simulink model "gm_DOA_rearanged"  (R2020b)
settings: Solver=ode4  StartTime=0.0  StopTime=0.25  RelTol=1e-3
undefined symbols (not defined in the file or in its folder): Coeff_han, FFT_LENGTH, Sampling_rate
libraries: dsphdlmathfun x4, dsphdlxfrm x4, simulink x1, hdlsllib x1
settings Model: Creator=tigro  LastModifiedBy=franc
settings OptimizationCC: BlockReduction=off  ConditionallyExecuteInputs=off  DefaultParameterBehavior=Inlined
settings DebuggingCC: AlgebraicLoopMsg=error  InheritedTsInSrcMsg=none  ParameterOverflowMsg=none
settings HardwareCC: ProdBitPerPointer=32  ProdBitPerSizeT=32  ProdBitPerPtrDiffT=32  ProdLargestAtomicFloat=None  ProdIntDivRoundTo=Undefined  ProdEndianess=Unspecified  ProdWordSize=32  ProdHWDeviceType=ASIC/FPGA->ASIC/FPGA  TargetBitPerPointer=64  TargetBitPerSizeT=64  TargetBitPerPtrDiffT=64  TargetLongLongMode=on  TargetIntDivRoundTo=Zero  TargetEndianess=LittleEndian  TargetWordSize=64  TargetHWDeviceType=Custom Processor->MATLAB Host Computer  ProdEqTarget=off

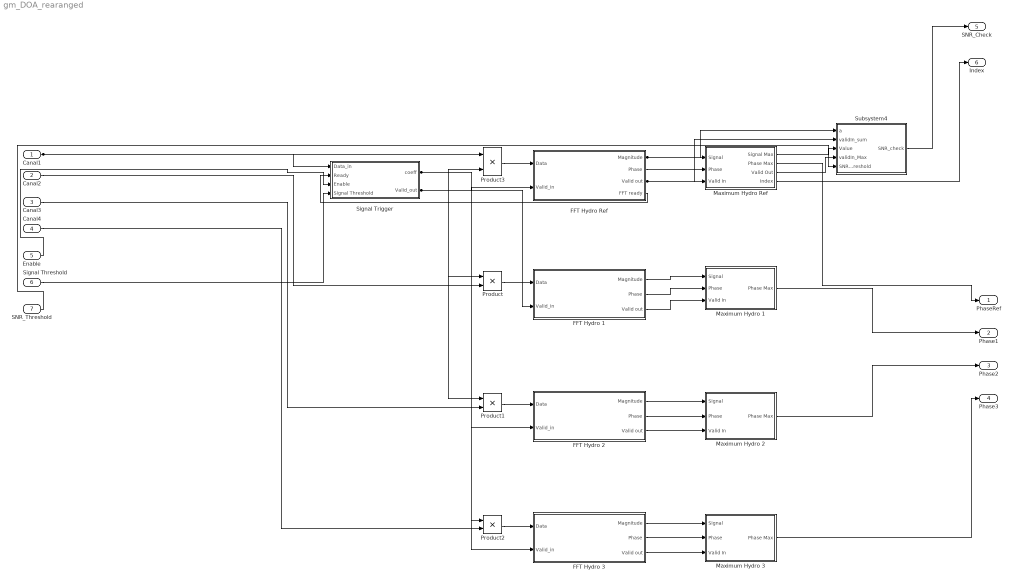
== system gm_DOA_rearanged ==
  Canal1 : Inport  OutDataTypeStr=uint16  PortDimensions=1  SampleTime=3.90625e-06
  Canal2 : Inport  Port=2  OutDataTypeStr=uint16  PortDimensions=1  SampleTime=3.90625e-06
  Canal3 : Inport  Port=3  OutDataTypeStr=uint16  PortDimensions=1  SampleTime=3.90625e-06
  Canal4 : Inport  Port=4  OutDataTypeStr=uint16  PortDimensions=1  SampleTime=3.90625e-06
  Enable : Inport  Port=5  OutDataTypeStr=boolean  PortDimensions=1  SampleTime=3.90625e-06
  Signal Threshold : Inport  Port=6  OutDataTypeStr=uint16  PortDimensions=1  SampleTime=3.90625e-06
  SNR_Threshold : Inport  Port=7  OutDataTypeStr=uint16  PortDimensions=1  SampleTime=3.90625e-06
  FFT Hydro 1 : Subsystem
  FFT Hydro 2 : Subsystem
  FFT Hydro 3 : Subsystem
  FFT Hydro Ref : Subsystem
  Maximum Hydro 1 : Subsystem
  Maximum Hydro 2 : Subsystem
  Maximum Hydro 3 : Subsystem
  Maximum Hydro Ref : Subsystem
  Product{,1..3} (4 alike) : Product
  Signal Trigger : Subsystem
  Subsystem4 : Subsystem
  PhaseRef : Outport
  Phase1 : Outport  Port=2
  Phase2 : Outport  Port=3
  Phase3 : Outport  Port=4
  SNR_Check : Outport  Port=5
  Index : Outport  Port=6
  wires:
  Canal1/1 -> Signal Trigger/1(Data_in), Product3/1
  Canal2/1 -> Product/2
  Canal3/1 -> Product1/2
  Canal4/1 -> Product2/2
  Enable/1 -> Signal Trigger/3(Enable)
  Signal Threshold/1 -> Signal Trigger/4(Signal Threshold)
  SNR_Threshold/1 -> Subsystem4/5(SNR_Threshold)
  FFT Hydro 1/1(Magnitude) -> Maximum Hydro 1/1(Signal)
  FFT Hydro 1/2(Phase) -> Maximum Hydro 1/2(Phase)
  FFT Hydro 1/3(Valid out) -> Maximum Hydro 1/3(Valid In)
  FFT Hydro 2/1(Magnitude) -> Maximum Hydro 2/1(Signal)
  FFT Hydro 2/2(Phase) -> Maximum Hydro 2/2(Phase)
  FFT Hydro 2/3(Valid out) -> Maximum Hydro 2/3(Valid In)
  FFT Hydro 3/1(Magnitude) -> Maximum Hydro 3/1(Signal)
  FFT Hydro 3/2(Phase) -> Maximum Hydro 3/2(Phase)
  FFT Hydro 3/3(Valid out) -> Maximum Hydro 3/3(Valid In)
  FFT Hydro Ref/1(Magnitude) -> Subsystem4/1(a), Maximum Hydro Ref/1(Signal)
  FFT Hydro Ref/2(Phase) -> Maximum Hydro Ref/2(Phase)
  FFT Hydro Ref/3(Valid out) -> Maximum Hydro Ref/3(Valid In), Subsystem4/2(validIn_sum)
  Maximum Hydro 1/1(Phase Max) -> Phase1/1
  Maximum Hydro 2/1(Phase Max) -> Phase2/1
  Maximum Hydro 3/1(Phase Max) -> Phase3/1
  Maximum Hydro Ref/1(Signal Max) -> Subsystem4/3(" Value")
  Maximum Hydro Ref/2(Phase Max) -> PhaseRef/1
  Maximum Hydro Ref/3(Valid Out) -> Subsystem4/4(validIn_Max)
  Maximum Hydro Ref/4(Index) -> Index/1
  Product/1 -> FFT Hydro 1/1(Data)
  Product1/1 -> FFT Hydro 2/1(Data)
  Product2/1 -> FFT Hydro 3/1(Data)
  Signal Trigger/1(coeff) -> Product2/1, Product1/1, Product/1, Product3/2
  Signal Trigger/2(Valid_out) -> FFT Hydro 1/2(Valid_in), FFT Hydro 3/2(Valid_in), FFT Hydro 2/2(Valid_in), FFT Hydro Ref/2(Valid_in)
  Subsystem4/1(SNR_check) -> SNR_Check/1
  Product3/1 -> FFT Hydro Ref/1(Data)
  FFT Hydro Ref/4(FFT ready) -> Signal Trigger/2(Ready)

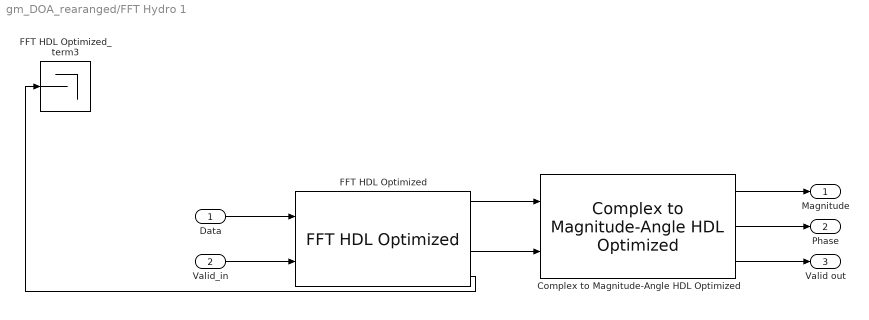
== system gm_DOA_rearanged/FFT Hydro 1 ==
  Data : Inport  OutDataTypeStr=fixdt(0, 25, 8)  PortDimensions=1  SampleTime=3.90625e-06
  Valid_in : Inport  Port=2  OutDataTypeStr=boolean  PortDimensions=1  SampleTime=3.90625e-06
  Complex to Magnitude-Angle HDL Optimized : dsphdlmathfun/Complex to Magnitude-Angle HDL Optimized  NumIterationsSource=Property  NumIterations=12  OutputFormat=Magnitude and angle  AngleFormat=Radians  ScaleOutput=on  SimulateUsing=Code generation
      settings: SourceProductBaseCode=DS
  FFT HDL Optimized : dsphdlxfrm/FFT HDL Optimized  FFTLength=FFT_LENGTH  Architecture=Burst Radix 2  ComplexMultiplication=Use 3 multipliers and 5 adders  BitReversedOutput=off  BitReversedInput=off  Normalize=on  SimulateUsing=Code generation  RoundingMethod=Floor  ResetInputPort=off  StartOutputPort=off  EndOutputPort=on
      settings: SourceProductBaseCode=DS
  FFT HDL Optimized_term3 : Terminator
  Magnitude : Outport
  Phase : Outport  Port=2
  Valid out : Outport  Port=3
  wires:
  Data/1 -> FFT HDL Optimized/1
  Valid_in/1 -> FFT HDL Optimized/2
  Complex to Magnitude-Angle HDL Optimized/1 -> Magnitude/1
  Complex to Magnitude-Angle HDL Optimized/2 -> Phase/1
  Complex to Magnitude-Angle HDL Optimized/3 -> Valid out/1
  FFT HDL Optimized/1 -> Complex to Magnitude-Angle HDL Optimized/1
  FFT HDL Optimized/3 -> Complex to Magnitude-Angle HDL Optimized/2
  FFT HDL Optimized/4 -> FFT HDL Optimized_term3/1

== system gm_DOA_rearanged/FFT Hydro 2 ==
  Data : Inport  OutDataTypeStr=fixdt(0, 25, 8)  PortDimensions=1  SampleTime=3.90625e-06
  Valid_in : Inport  Port=2  OutDataTypeStr=boolean  PortDimensions=1  SampleTime=3.90625e-06
  Complex to Magnitude-Angle HDL Optimized : dsphdlmathfun/Complex to Magnitude-Angle HDL Optimized  NumIterationsSource=Property  NumIterations=12  OutputFormat=Magnitude and angle  AngleFormat=Radians  ScaleOutput=on  SimulateUsing=Code generation
      settings: SourceProductBaseCode=DS
  FFT HDL Optimized : dsphdlxfrm/FFT HDL Optimized  FFTLength=FFT_LENGTH  Architecture=Burst Radix 2  ComplexMultiplication=Use 3 multipliers and 5 adders  BitReversedOutput=off  BitReversedInput=off  Normalize=on  SimulateUsing=Code generation  RoundingMethod=Floor  ResetInputPort=off  StartOutputPort=off  EndOutputPort=off
      settings: SourceProductBaseCode=DS
  Magnitude : Outport
  Phase : Outport  Port=2
  Valid out : Outport  Port=3
  wires:
  Data/1 -> FFT HDL Optimized/1
  Valid_in/1 -> FFT HDL Optimized/2
  Complex to Magnitude-Angle HDL Optimized/1 -> Magnitude/1
  Complex to Magnitude-Angle HDL Optimized/2 -> Phase/1
  Complex to Magnitude-Angle HDL Optimized/3 -> Valid out/1
  FFT HDL Optimized/1 -> Complex to Magnitude-Angle HDL Optimized/1
  FFT HDL Optimized/2 -> Complex to Magnitude-Angle HDL Optimized/2

== system gm_DOA_rearanged/FFT Hydro 3 ==
  Data : Inport  OutDataTypeStr=fixdt(0, 25, 8)  PortDimensions=1  SampleTime=3.90625e-06
  Valid_in : Inport  Port=2  OutDataTypeStr=boolean  PortDimensions=1  SampleTime=3.90625e-06
  Complex to Magnitude-Angle HDL Optimized : dsphdlmathfun/Complex to Magnitude-Angle HDL Optimized  NumIterationsSource=Property  NumIterations=12  OutputFormat=Magnitude and angle  AngleFormat=Radians  ScaleOutput=on  SimulateUsing=Code generation
      settings: SourceProductBaseCode=DS
  FFT HDL Optimized : dsphdlxfrm/FFT HDL Optimized  FFTLength=FFT_LENGTH  Architecture=Burst Radix 2  ComplexMultiplication=Use 3 multipliers and 5 adders  BitReversedOutput=off  BitReversedInput=off  Normalize=on  SimulateUsing=Code generation  RoundingMethod=Floor  ResetInputPort=off  StartOutputPort=off  EndOutputPort=off
      settings: SourceProductBaseCode=DS
  Magnitude : Outport
  Phase : Outport  Port=2
  Valid out : Outport  Port=3
  wires:
  Data/1 -> FFT HDL Optimized/1
  Valid_in/1 -> FFT HDL Optimized/2
  Complex to Magnitude-Angle HDL Optimized/1 -> Magnitude/1
  Complex to Magnitude-Angle HDL Optimized/2 -> Phase/1
  Complex to Magnitude-Angle HDL Optimized/3 -> Valid out/1
  FFT HDL Optimized/1 -> Complex to Magnitude-Angle HDL Optimized/1
  FFT HDL Optimized/2 -> Complex to Magnitude-Angle HDL Optimized/2

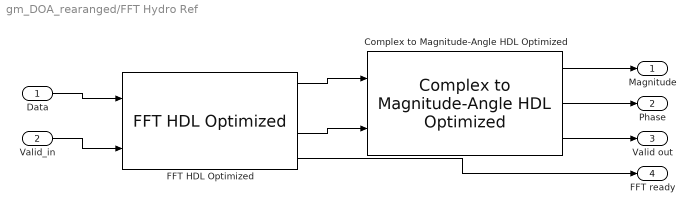
== system gm_DOA_rearanged/FFT Hydro Ref ==
  Data : Inport  OutDataTypeStr=fixdt(0, 25, 8)  PortDimensions=1  SampleTime=3.90625e-06
  Valid_in : Inport  Port=2  OutDataTypeStr=boolean  PortDimensions=1  SampleTime=3.90625e-06
  Complex to Magnitude-Angle HDL Optimized : dsphdlmathfun/Complex to Magnitude-Angle HDL Optimized  NumIterationsSource=Property  NumIterations=12  OutputFormat=Magnitude and angle  AngleFormat=Radians  ScaleOutput=on  SimulateUsing=Code generation
      settings: SourceProductBaseCode=DS
  FFT HDL Optimized : dsphdlxfrm/FFT HDL Optimized  FFTLength=FFT_LENGTH  Architecture=Burst Radix 2  ComplexMultiplication=Use 3 multipliers and 5 adders  BitReversedOutput=off  BitReversedInput=off  Normalize=on  SimulateUsing=Code generation  RoundingMethod=Floor  ResetInputPort=off  StartOutputPort=off  EndOutputPort=on
      settings: SourceProductBaseCode=DS
  Magnitude : Outport
  Phase : Outport  Port=2
  Valid out : Outport  Port=3
  FFT ready : Outport  Port=4
  wires:
  Data/1 -> FFT HDL Optimized/1
  Valid_in/1 -> FFT HDL Optimized/2
  Complex to Magnitude-Angle HDL Optimized/1 -> Magnitude/1
  Complex to Magnitude-Angle HDL Optimized/2 -> Phase/1
  Complex to Magnitude-Angle HDL Optimized/3 -> Valid out/1
  FFT HDL Optimized/1 -> Complex to Magnitude-Angle HDL Optimized/1
  FFT HDL Optimized/3 -> Complex to Magnitude-Angle HDL Optimized/2
  FFT HDL Optimized/4 -> FFT ready/1

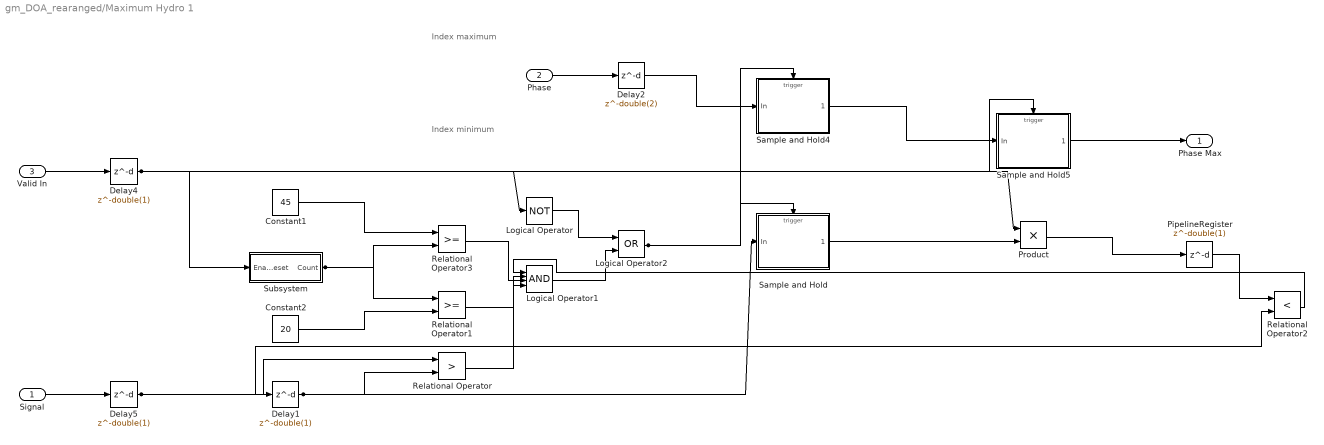
== system gm_DOA_rearanged/Maximum Hydro 1 ==
  note: Index maximum
  note: Index minimum
  Signal : Inport  OutDataTypeStr=fixdt(1, 27, 8)  PortDimensions=1  SampleTime=3.90625e-06
  Phase : Inport  Port=2  OutDataTypeStr=fixdt(1, 29, 26)  PortDimensions=1  SampleTime=3.90625e-06
  Valid In : Inport  Port=3  OutDataTypeStr=boolean  PortDimensions=1  SampleTime=3.90625e-06
  Constant1 : Constant  Value=45  OutDataTypeStr=fixdt(0, 6, 0)  SampleTime=3.90625e-06
  Constant2 : Constant  Value=20  OutDataTypeStr=fixdt(0, 6, 1)  SampleTime=3.90625e-06
  Delay1 : Delay  DelayLength=double(1)  InitialCondition=0  SampleTime=3.90625e-06
  Delay2 : Delay  DelayLength=double(2)  InitialCondition=0  SampleTime=3.90625e-06
  Delay4 : Delay  DelayLength=double(1)  InitialCondition=0  SampleTime=3.90625e-06
  Delay5 : Delay  DelayLength=double(1)  InitialCondition=0  SampleTime=3.90625e-06
  Logical Operator : Logic  Operator=NOT  Inputs=1  AllPortsSameDT=off  OutDataTypeStr=boolean  SampleTime=3.90625e-06
  Logical Operator1 : Logic  Inputs=4  AllPortsSameDT=off  OutDataTypeStr=boolean  SampleTime=3.90625e-06
  Logical Operator2 : Logic  Operator=OR  AllPortsSameDT=off  OutDataTypeStr=boolean  SampleTime=3.90625e-06
  PipelineRegister : Delay  DelayLength=double(1)  InitialCondition=0  SampleTime=3.90625e-06
  Product : Product  Inputs=**  OutDataTypeStr=fixdt(1, 27, 8)  SampleTime=3.90625e-06
  Relational Operator : RelationalOperator  Operator=>  OutDataTypeStr=boolean  SampleTime=3.90625e-06  RndMeth=Nearest
  Relational Operator1 : RelationalOperator  OutDataTypeStr=boolean  SampleTime=3.90625e-06  RndMeth=Nearest
  Relational Operator2 : RelationalOperator  Operator=<  OutDataTypeStr=boolean  SampleTime=3.90625e-06  RndMeth=Nearest
  Relational Operator3 : RelationalOperator  OutDataTypeStr=boolean  SampleTime=3.90625e-06  RndMeth=Nearest
  Sample and Hold : Subsystem  mask(Sample and Hold){trig=Falling edge, initCond=double(0), latchinput=off}
      mask prompts: trig "Trigger type:"; initCond "Initial condition:"; latchinput "Latch (buffer) input"
      mask help: Sample and hold the input signal. If Latch (buffer) input is selected, then this block produces the value of the input from the previous time step.
      mask init:
      | switch trig
      | case 1, s='rising';
      | case 2, s='falling';
      | case 3, s='either';
      | end
      | set_param([gcb '/Trigger'],'triggertype',s);
      | if (latchinput == 1)
      | 	set_param([gcb '/In'],'latchinput','on');
      | else
      | 	set_param([gcb '/In'],'latchinput','off');
      | end
      mask Help: eval('blocksethelp');
      mask TypeOptions trig: Rising edge | Falling edge | Either edge
      mask Display: disp('S/H')
  Sample and Hold4 : Subsystem  mask(Sample and Hold){trig=Falling edge, initCond=double(0), latchinput=off}
      mask prompts: trig "Trigger type:"; initCond "Initial condition:"; latchinput "Latch (buffer) input"
      mask help: Sample and hold the input signal. If Latch (buffer) input is selected, then this block produces the value of the input from the previous time step.
      mask init: same as gm_DOA_rearanged/Maximum Hydro 1/Sample and Hold
      mask Help: eval('blocksethelp');
      mask TypeOptions trig: Rising edge | Falling edge | Either edge
      mask Display: disp('S/H')
  Sample and Hold5 : Subsystem  mask(Sample and Hold){trig=Falling edge, initCond=double(0), latchinput=off}
      mask prompts: trig "Trigger type:"; initCond "Initial condition:"; latchinput "Latch (buffer) input"
      mask help: Sample and hold the input signal. If Latch (buffer) input is selected, then this block produces the value of the input from the previous time step.
      mask init: same as gm_DOA_rearanged/Maximum Hydro 1/Sample and Hold
      mask Help: eval('blocksethelp');
      mask TypeOptions trig: Rising edge | Falling edge | Either edge
      mask Display: disp('S/H')
  Subsystem : Subsystem
  Phase Max : Outport  VectorParamsAs1DForOutWhenUnconnected=off
  wires:
  Signal/1 -> Delay5/1
  Phase/1 -> Delay2/1
  Valid In/1 -> Delay4/1
  Constant1/1 -> Relational Operator3/1
  Constant2/1 -> Relational Operator1/2
  Delay1/1 -> Relational Operator/2, Sample and Hold/1(In)
  Delay2/1 -> Sample and Hold4/1(In)
  Delay4/1 -> Logical Operator/1, Sample and Hold5/Trigger, Subsystem/1(Enable/Reset), Product/1
  Delay5/1 -> Relational Operator/1, Delay1/1, Relational Operator2/2
  Logical Operator/1 -> Logical Operator2/1
  Logical Operator2/1 -> Sample and Hold4/Trigger, Sample and Hold/Trigger
  Relational Operator/1 -> Logical Operator1/2
  Relational Operator1/1 -> Logical Operator1/4
  Relational Operator3/1 -> Logical Operator1/3
  Sample and Hold4/1(" ") -> Sample and Hold5/1(In)
  Sample and Hold5/1(" ") -> Phase Max/1
  Subsystem/1(Count) -> Relational Operator3/2, Relational Operator1/1
  Sample and Hold/1(" ") -> Product/2
  PipelineRegister/1 -> Relational Operator2/1
  Relational Operator2/1 -> Logical Operator1/1
  Logical Operator1/1 -> Logical Operator2/2
  Product/1 -> PipelineRegister/1

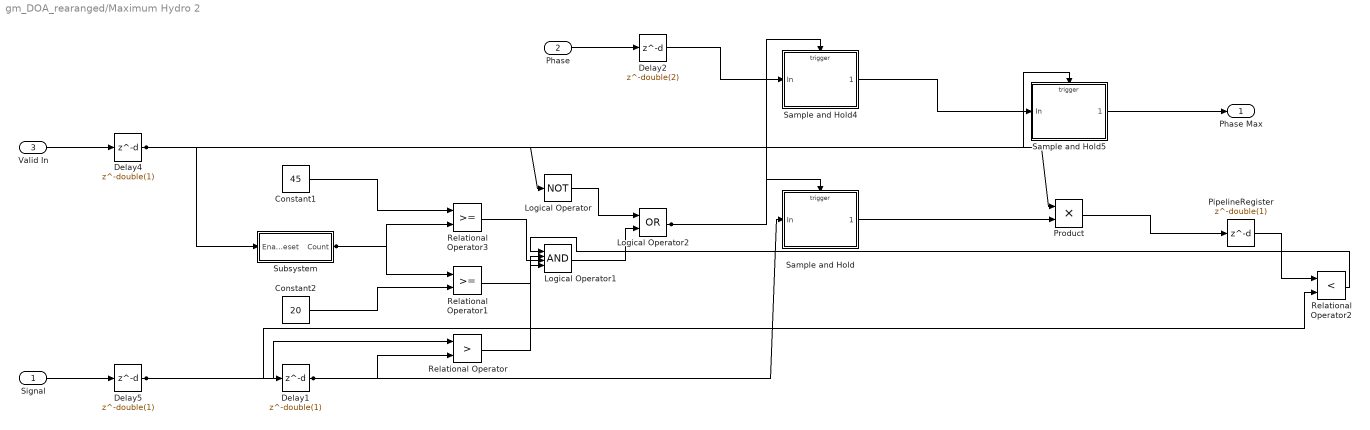
== system gm_DOA_rearanged/Maximum Hydro 2 ==
  Signal : Inport  OutDataTypeStr=fixdt(1, 27, 8)  PortDimensions=1  SampleTime=3.90625e-06
  Phase : Inport  Port=2  OutDataTypeStr=fixdt(1, 29, 26)  PortDimensions=1  SampleTime=3.90625e-06
  Valid In : Inport  Port=3  OutDataTypeStr=boolean  PortDimensions=1  SampleTime=3.90625e-06
  Constant1 : Constant  Value=45  OutDataTypeStr=fixdt(0, 6, 0)  SampleTime=3.90625e-06
  Constant2 : Constant  Value=20  OutDataTypeStr=fixdt(0, 6, 1)  SampleTime=3.90625e-06
  Delay1 : Delay  DelayLength=double(1)  InitialCondition=0  SampleTime=3.90625e-06
  Delay2 : Delay  DelayLength=double(2)  InitialCondition=0  SampleTime=3.90625e-06
  Delay4 : Delay  DelayLength=double(1)  InitialCondition=0  SampleTime=3.90625e-06
  Delay5 : Delay  DelayLength=double(1)  InitialCondition=0  SampleTime=3.90625e-06
  Logical Operator : Logic  Operator=NOT  Inputs=1  AllPortsSameDT=off  OutDataTypeStr=boolean  SampleTime=3.90625e-06
  Logical Operator1 : Logic  Inputs=4  AllPortsSameDT=off  OutDataTypeStr=boolean  SampleTime=3.90625e-06
  Logical Operator2 : Logic  Operator=OR  AllPortsSameDT=off  OutDataTypeStr=boolean  SampleTime=3.90625e-06
  PipelineRegister : Delay  DelayLength=double(1)  InitialCondition=0  SampleTime=3.90625e-06
  Product : Product  Inputs=**  OutDataTypeStr=fixdt(1, 27, 8)  SampleTime=3.90625e-06
  Relational Operator : RelationalOperator  Operator=>  OutDataTypeStr=boolean  SampleTime=3.90625e-06  RndMeth=Nearest
  Relational Operator1 : RelationalOperator  OutDataTypeStr=boolean  SampleTime=3.90625e-06  RndMeth=Nearest
  Relational Operator2 : RelationalOperator  Operator=<  OutDataTypeStr=boolean  SampleTime=3.90625e-06  RndMeth=Nearest
  Relational Operator3 : RelationalOperator  OutDataTypeStr=boolean  SampleTime=3.90625e-06  RndMeth=Nearest
  Sample and Hold : Subsystem  mask(Sample and Hold){trig=Falling edge, initCond=double(0), latchinput=off}
      mask prompts: trig "Trigger type:"; initCond "Initial condition:"; latchinput "Latch (buffer) input"
      mask help: Sample and hold the input signal. If Latch (buffer) input is selected, then this block produces the value of the input from the previous time step.
      mask init: same as gm_DOA_rearanged/Maximum Hydro 1/Sample and Hold
      mask Help: eval('blocksethelp');
      mask TypeOptions trig: Rising edge | Falling edge | Either edge
      mask Display: disp('S/H')
  Sample and Hold4 : Subsystem  mask(Sample and Hold){trig=Falling edge, initCond=double(0), latchinput=off}
      mask prompts: trig "Trigger type:"; initCond "Initial condition:"; latchinput "Latch (buffer) input"
      mask help: Sample and hold the input signal. If Latch (buffer) input is selected, then this block produces the value of the input from the previous time step.
      mask init: same as gm_DOA_rearanged/Maximum Hydro 1/Sample and Hold
      mask Help: eval('blocksethelp');
      mask TypeOptions trig: Rising edge | Falling edge | Either edge
      mask Display: disp('S/H')
  Sample and Hold5 : Subsystem  mask(Sample and Hold){trig=Falling edge, initCond=double(0), latchinput=off}
      mask prompts: trig "Trigger type:"; initCond "Initial condition:"; latchinput "Latch (buffer) input"
      mask help: Sample and hold the input signal. If Latch (buffer) input is selected, then this block produces the value of the input from the previous time step.
      mask init: same as gm_DOA_rearanged/Maximum Hydro 1/Sample and Hold
      mask Help: eval('blocksethelp');
      mask TypeOptions trig: Rising edge | Falling edge | Either edge
      mask Display: disp('S/H')
  Subsystem : Subsystem
  Phase Max : Outport  VectorParamsAs1DForOutWhenUnconnected=off
  wires:
  Signal/1 -> Delay5/1
  Phase/1 -> Delay2/1
  Valid In/1 -> Delay4/1
  Constant1/1 -> Relational Operator3/1
  Constant2/1 -> Relational Operator1/2
  Delay1/1 -> Relational Operator/2, Sample and Hold/1(In)
  Delay2/1 -> Sample and Hold4/1(In)
  Delay4/1 -> Logical Operator/1, Sample and Hold5/Trigger, Subsystem/1(Enable/Reset), Product/1
  Delay5/1 -> Relational Operator/1, Delay1/1, Relational Operator2/2
  Logical Operator/1 -> Logical Operator2/1
  Logical Operator2/1 -> Sample and Hold4/Trigger, Sample and Hold/Trigger
  Relational Operator/1 -> Logical Operator1/2
  Relational Operator1/1 -> Logical Operator1/4
  Relational Operator3/1 -> Logical Operator1/3
  Sample and Hold4/1(" ") -> Sample and Hold5/1(In)
  Sample and Hold5/1(" ") -> Phase Max/1
  Subsystem/1(Count) -> Relational Operator3/2, Relational Operator1/1
  Sample and Hold/1(" ") -> Product/2
  PipelineRegister/1 -> Relational Operator2/1
  Relational Operator2/1 -> Logical Operator1/1
  Logical Operator1/1 -> Logical Operator2/2
  Product/1 -> PipelineRegister/1

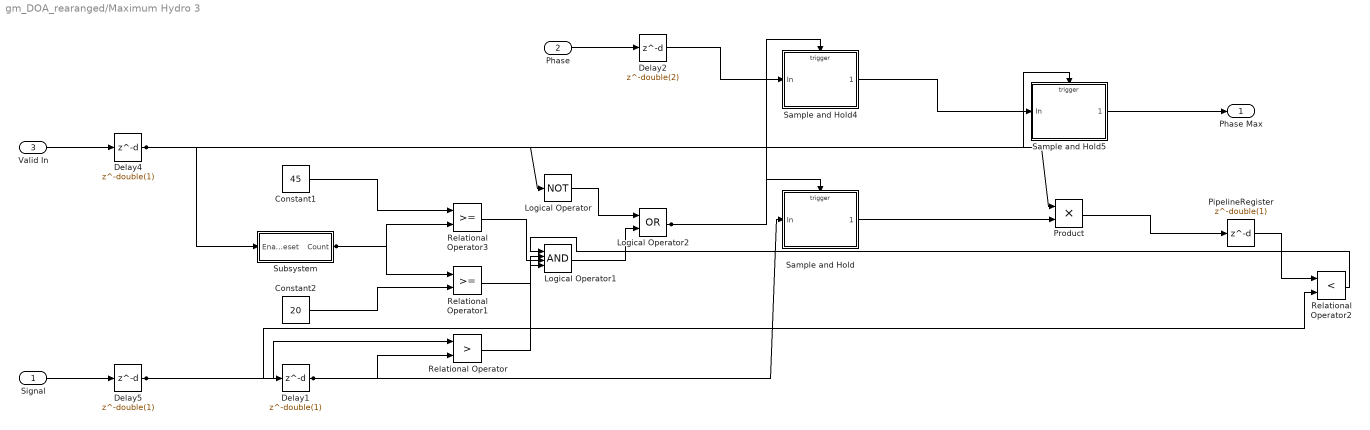
== system gm_DOA_rearanged/Maximum Hydro 3 ==
  Signal : Inport  OutDataTypeStr=fixdt(1, 27, 8)  PortDimensions=1  SampleTime=3.90625e-06
  Phase : Inport  Port=2  OutDataTypeStr=fixdt(1, 29, 26)  PortDimensions=1  SampleTime=3.90625e-06
  Valid In : Inport  Port=3  OutDataTypeStr=boolean  PortDimensions=1  SampleTime=3.90625e-06
  Constant1 : Constant  Value=45  OutDataTypeStr=fixdt(0, 6, 0)  SampleTime=3.90625e-06
  Constant2 : Constant  Value=20  OutDataTypeStr=fixdt(0, 6, 1)  SampleTime=3.90625e-06
  Delay1 : Delay  DelayLength=double(1)  InitialCondition=0  SampleTime=3.90625e-06
  Delay2 : Delay  DelayLength=double(2)  InitialCondition=0  SampleTime=3.90625e-06
  Delay4 : Delay  DelayLength=double(1)  InitialCondition=0  SampleTime=3.90625e-06
  Delay5 : Delay  DelayLength=double(1)  InitialCondition=0  SampleTime=3.90625e-06
  Logical Operator : Logic  Operator=NOT  Inputs=1  AllPortsSameDT=off  OutDataTypeStr=boolean  SampleTime=3.90625e-06
  Logical Operator1 : Logic  Inputs=4  AllPortsSameDT=off  OutDataTypeStr=boolean  SampleTime=3.90625e-06
  Logical Operator2 : Logic  Operator=OR  AllPortsSameDT=off  OutDataTypeStr=boolean  SampleTime=3.90625e-06
  PipelineRegister : Delay  DelayLength=double(1)  InitialCondition=0  SampleTime=3.90625e-06
  Product : Product  Inputs=**  OutDataTypeStr=fixdt(1, 27, 8)  SampleTime=3.90625e-06
  Relational Operator : RelationalOperator  Operator=>  OutDataTypeStr=boolean  SampleTime=3.90625e-06  RndMeth=Nearest
  Relational Operator1 : RelationalOperator  OutDataTypeStr=boolean  SampleTime=3.90625e-06  RndMeth=Nearest
  Relational Operator2 : RelationalOperator  Operator=<  OutDataTypeStr=boolean  SampleTime=3.90625e-06  RndMeth=Nearest
  Relational Operator3 : RelationalOperator  OutDataTypeStr=boolean  SampleTime=3.90625e-06  RndMeth=Nearest
  Sample and Hold : Subsystem  mask(Sample and Hold){trig=Falling edge, initCond=double(0), latchinput=off}
      mask prompts: trig "Trigger type:"; initCond "Initial condition:"; latchinput "Latch (buffer) input"
      mask help: Sample and hold the input signal. If Latch (buffer) input is selected, then this block produces the value of the input from the previous time step.
      mask init: same as gm_DOA_rearanged/Maximum Hydro 1/Sample and Hold
      mask Help: eval('blocksethelp');
      mask TypeOptions trig: Rising edge | Falling edge | Either edge
      mask Display: disp('S/H')
  Sample and Hold4 : Subsystem  mask(Sample and Hold){trig=Falling edge, initCond=double(0), latchinput=off}
      mask prompts: trig "Trigger type:"; initCond "Initial condition:"; latchinput "Latch (buffer) input"
      mask help: Sample and hold the input signal. If Latch (buffer) input is selected, then this block produces the value of the input from the previous time step.
      mask init: same as gm_DOA_rearanged/Maximum Hydro 1/Sample and Hold
      mask Help: eval('blocksethelp');
      mask TypeOptions trig: Rising edge | Falling edge | Either edge
      mask Display: disp('S/H')
  Sample and Hold5 : Subsystem  mask(Sample and Hold){trig=Falling edge, initCond=double(0), latchinput=off}
      mask prompts: trig "Trigger type:"; initCond "Initial condition:"; latchinput "Latch (buffer) input"
      mask help: Sample and hold the input signal. If Latch (buffer) input is selected, then this block produces the value of the input from the previous time step.
      mask init: same as gm_DOA_rearanged/Maximum Hydro 1/Sample and Hold
      mask Help: eval('blocksethelp');
      mask TypeOptions trig: Rising edge | Falling edge | Either edge
      mask Display: disp('S/H')
  Subsystem : Subsystem
  Phase Max : Outport  VectorParamsAs1DForOutWhenUnconnected=off
  wires:
  Signal/1 -> Delay5/1
  Phase/1 -> Delay2/1
  Valid In/1 -> Delay4/1
  Constant1/1 -> Relational Operator3/1
  Constant2/1 -> Relational Operator1/2
  Delay1/1 -> Relational Operator/2, Sample and Hold/1(In)
  Delay2/1 -> Sample and Hold4/1(In)
  Delay4/1 -> Logical Operator/1, Sample and Hold5/Trigger, Subsystem/1(Enable/Reset), Product/1
  Delay5/1 -> Relational Operator/1, Delay1/1, Relational Operator2/2
  Logical Operator/1 -> Logical Operator2/1
  Logical Operator2/1 -> Sample and Hold4/Trigger, Sample and Hold/Trigger
  Relational Operator/1 -> Logical Operator1/2
  Relational Operator1/1 -> Logical Operator1/4
  Relational Operator3/1 -> Logical Operator1/3
  Sample and Hold4/1(" ") -> Sample and Hold5/1(In)
  Sample and Hold5/1(" ") -> Phase Max/1
  Subsystem/1(Count) -> Relational Operator3/2, Relational Operator1/1
  Sample and Hold/1(" ") -> Product/2
  PipelineRegister/1 -> Relational Operator2/1
  Relational Operator2/1 -> Logical Operator1/1
  Logical Operator1/1 -> Logical Operator2/2
  Product/1 -> PipelineRegister/1

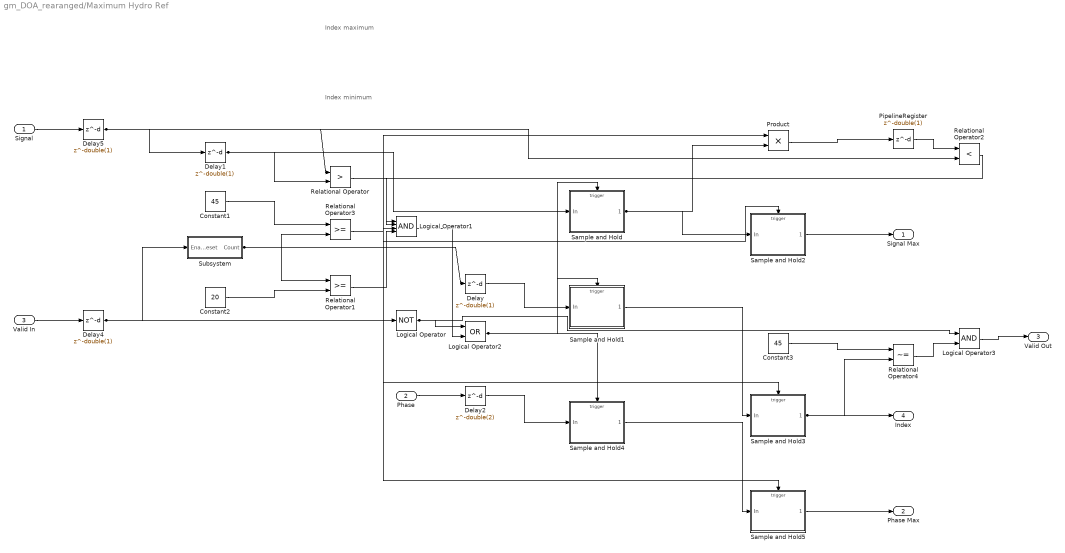
== system gm_DOA_rearanged/Maximum Hydro Ref ==
  note: Index maximum
  note: Index minimum
  Signal : Inport  OutDataTypeStr=fixdt(1, 27, 8)  PortDimensions=1  SampleTime=3.90625e-06
  Phase : Inport  Port=2  OutDataTypeStr=fixdt(1, 29, 26)  PortDimensions=1  SampleTime=3.90625e-06
  Valid In : Inport  Port=3  OutDataTypeStr=boolean  PortDimensions=1  SampleTime=3.90625e-06
  Constant1 : Constant  Value=45  OutDataTypeStr=fixdt(0, 6, 0)  SampleTime=3.90625e-06
  Constant2 : Constant  Value=20  OutDataTypeStr=fixdt(0, 6, 1)  SampleTime=3.90625e-06
  Constant3 : Constant  Value=45  OutDataTypeStr=fixdt(0, 6, 0)  SampleTime=3.90625e-06
  Delay{,1,4..5} (4 alike) : Delay  DelayLength=double(1)  InitialCondition=0  SampleTime=3.90625e-06
  Delay2 : Delay  DelayLength=double(2)  InitialCondition=0  SampleTime=3.90625e-06
  Logical Operator : Logic  Operator=NOT  Inputs=1  AllPortsSameDT=off  OutDataTypeStr=boolean  SampleTime=3.90625e-06
  Logical Operator1 : Logic  Inputs=4  AllPortsSameDT=off  OutDataTypeStr=boolean  SampleTime=3.90625e-06
  Logical Operator2 : Logic  Operator=OR  AllPortsSameDT=off  OutDataTypeStr=boolean  SampleTime=3.90625e-06
  Logical Operator3 : Logic  AllPortsSameDT=off  OutDataTypeStr=boolean  SampleTime=3.90625e-06
  PipelineRegister : Delay  DelayLength=double(1)  InitialCondition=0  SampleTime=3.90625e-06
  Product : Product  Inputs=**  OutDataTypeStr=fixdt(1, 27, 8)  SampleTime=3.90625e-06
  Relational Operator : RelationalOperator  Operator=>  OutDataTypeStr=boolean  SampleTime=3.90625e-06  RndMeth=Nearest
  Relational Operator1 : RelationalOperator  OutDataTypeStr=boolean  SampleTime=3.90625e-06  RndMeth=Nearest
  Relational Operator2 : RelationalOperator  Operator=<  OutDataTypeStr=boolean  SampleTime=3.90625e-06  RndMeth=Nearest
  Relational Operator3 : RelationalOperator  OutDataTypeStr=boolean  SampleTime=3.90625e-06  RndMeth=Nearest
  Relational Operator4 : RelationalOperator  Operator=~=  OutDataTypeStr=boolean  SampleTime=3.90625e-06  RndMeth=Nearest
  Sample and Hold : Subsystem  mask(Sample and Hold){trig=Falling edge, initCond=double(0), latchinput=off}
      mask prompts: trig "Trigger type:"; initCond "Initial condition:"; latchinput "Latch (buffer) input"
      mask help: Sample and hold the input signal. If Latch (buffer) input is selected, then this block produces the value of the input from the previous time step.
      mask init: same as gm_DOA_rearanged/Maximum Hydro 1/Sample and Hold
      mask Help: eval('blocksethelp');
      mask TypeOptions trig: Rising edge | Falling edge | Either edge
      mask Display: disp('S/H')
  Sample and Hold1 : Subsystem  mask(Sample and Hold){trig=Falling edge, initCond=double(0), latchinput=off}
      mask prompts: trig "Trigger type:"; initCond "Initial condition:"; latchinput "Latch (buffer) input"
      mask help: Sample and hold the input signal. If Latch (buffer) input is selected, then this block produces the value of the input from the previous time step.
      mask init: same as gm_DOA_rearanged/Maximum Hydro 1/Sample and Hold
      mask Help: eval('blocksethelp');
      mask TypeOptions trig: Rising edge | Falling edge | Either edge
      mask Display: disp('S/H')
  Sample and Hold2 : Subsystem  mask(Sample and Hold){trig=Falling edge, initCond=double(0), latchinput=off}
      mask prompts: trig "Trigger type:"; initCond "Initial condition:"; latchinput "Latch (buffer) input"
      mask help: Sample and hold the input signal. If Latch (buffer) input is selected, then this block produces the value of the input from the previous time step.
      mask init: same as gm_DOA_rearanged/Maximum Hydro 1/Sample and Hold
      mask Help: eval('blocksethelp');
      mask TypeOptions trig: Rising edge | Falling edge | Either edge
      mask Display: disp('S/H')
  Sample and Hold3 : Subsystem  mask(Sample and Hold){trig=Falling edge, initCond=double(0), latchinput=off}
      mask prompts: trig "Trigger type:"; initCond "Initial condition:"; latchinput "Latch (buffer) input"
      mask help: Sample and hold the input signal. If Latch (buffer) input is selected, then this block produces the value of the input from the previous time step.
      mask init: same as gm_DOA_rearanged/Maximum Hydro 1/Sample and Hold
      mask Help: eval('blocksethelp');
      mask TypeOptions trig: Rising edge | Falling edge | Either edge
      mask Display: disp('S/H')
  Sample and Hold4 : Subsystem  mask(Sample and Hold){trig=Falling edge, initCond=double(0), latchinput=off}
      mask prompts: trig "Trigger type:"; initCond "Initial condition:"; latchinput "Latch (buffer) input"
      mask help: Sample and hold the input signal. If Latch (buffer) input is selected, then this block produces the value of the input from the previous time step.
      mask init: same as gm_DOA_rearanged/Maximum Hydro 1/Sample and Hold
      mask Help: eval('blocksethelp');
      mask TypeOptions trig: Rising edge | Falling edge | Either edge
      mask Display: disp('S/H')
  Sample and Hold5 : Subsystem  mask(Sample and Hold){trig=Falling edge, initCond=double(0), latchinput=off}
      mask prompts: trig "Trigger type:"; initCond "Initial condition:"; latchinput "Latch (buffer) input"
      mask help: Sample and hold the input signal. If Latch (buffer) input is selected, then this block produces the value of the input from the previous time step.
      mask init: same as gm_DOA_rearanged/Maximum Hydro 1/Sample and Hold
      mask Help: eval('blocksethelp');
      mask TypeOptions trig: Rising edge | Falling edge | Either edge
      mask Display: disp('S/H')
  Subsystem : Subsystem
  Signal Max : Outport  VectorParamsAs1DForOutWhenUnconnected=off
  Phase Max : Outport  Port=2  VectorParamsAs1DForOutWhenUnconnected=off
  Valid Out : Outport  Port=3  VectorParamsAs1DForOutWhenUnconnected=off
  Index : Outport  Port=4  VectorParamsAs1DForOutWhenUnconnected=off
  wires:
  Signal/1 -> Delay5/1
  Phase/1 -> Delay2/1
  Valid In/1 -> Delay4/1
  Constant1/1 -> Relational Operator3/1
  Constant2/1 -> Relational Operator1/2
  Constant3/1 -> Relational Operator4/1
  Delay/1 -> Sample and Hold1/1(In)
  Delay1/1 -> Relational Operator/2, Sample and Hold/1(In)
  Delay2/1 -> Sample and Hold4/1(In)
  Delay4/1 -> Logical Operator/1, Sample and Hold2/Trigger, Sample and Hold3/Trigger, Sample and Hold5/Trigger, Subsystem/1(Enable/Reset), Product/1
  Delay5/1 -> Relational Operator/1, Delay1/1, Relational Operator2/2
  Logical Operator/1 -> Logical Operator3/1, Logical Operator2/1
  Logical Operator2/1 -> Sample and Hold4/Trigger, Sample and Hold1/Trigger, Sample and Hold/Trigger
  Logical Operator3/1 -> Valid Out/1
  Relational Operator/1 -> Logical Operator1/2
  Relational Operator1/1 -> Logical Operator1/4
  Relational Operator3/1 -> Logical Operator1/3
  Relational Operator4/1 -> Logical Operator3/2
  Sample and Hold/1(" ") -> Sample and Hold2/1(In), Product/2
  Sample and Hold1/1(" ") -> Sample and Hold3/1(In)
  Sample and Hold2/1(" ") -> Signal Max/1
  Sample and Hold3/1(" ") -> Relational Operator4/2, Index/1
  Sample and Hold4/1(" ") -> Sample and Hold5/1(In)
  Sample and Hold5/1(" ") -> Phase Max/1
  Subsystem/1(Count) -> Relational Operator3/2, Relational Operator1/1, Delay/1
  PipelineRegister/1 -> Relational Operator2/1
  Relational Operator2/1 -> Logical Operator1/1
  Logical Operator1/1 -> Logical Operator2/2
  Product/1 -> PipelineRegister/1

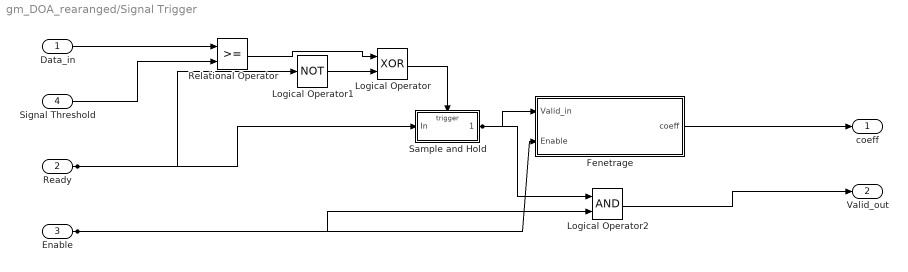
== system gm_DOA_rearanged/Signal Trigger ==
  Data_in : Inport  OutDataTypeStr=uint16  PortDimensions=1  SampleTime=3.90625e-06
  Ready : Inport  Port=2  OutDataTypeStr=boolean  PortDimensions=1  SampleTime=3.90625e-06
  Enable : Inport  Port=3  OutDataTypeStr=boolean  PortDimensions=1  SampleTime=3.90625e-06
  Signal Threshold : Inport  Port=4  OutDataTypeStr=uint16  PortDimensions=1  SampleTime=3.90625e-06
  Fenetrage : Subsystem
  Logical Operator : Logic  Operator=XOR  AllPortsSameDT=off  OutDataTypeStr=boolean
  Logical Operator1 : Logic  Operator=NOT  IconShape=distinctive  AllPortsSameDT=off  OutDataTypeStr=boolean
  Logical Operator2 : Logic  AllPortsSameDT=off  OutDataTypeStr=boolean
  Relational Operator : RelationalOperator  OutDataTypeStr=boolean  RndMeth=Nearest
  Sample and Hold : Subsystem  mask(Sample and Hold){trig=Rising edge, initCond=double(0), latchinput=off}
      mask prompts: trig "Trigger type:"; initCond "Initial condition:"; latchinput "Latch (buffer) input"
      mask help: Sample and hold the input signal. If Latch (buffer) input is selected, then this block produces the value of the input from the previous time step.
      mask init: same as gm_DOA_rearanged/Maximum Hydro 1/Sample and Hold
      mask Help: eval('blocksethelp');
      mask TypeOptions trig: Rising edge | Falling edge | Either edge
      mask Display: disp('S/H')
  coeff : Outport
  Valid_out : Outport  Port=2
  wires:
  Data_in/1 -> Relational Operator/1
  Ready/1 -> Logical Operator1/1, Sample and Hold/1(In)
  Enable/1 -> Logical Operator2/2, Fenetrage/2(Enable)
  Signal Threshold/1 -> Relational Operator/2
  Fenetrage/1(coeff) -> coeff/1
  Logical Operator/1 -> Sample and Hold/Trigger
  Logical Operator1/1 -> Logical Operator/2
  Logical Operator2/1 -> Valid_out/1
  Relational Operator/1 -> Logical Operator/1
  Sample and Hold/1(" ") -> Logical Operator2/1, Fenetrage/1(Valid_in)

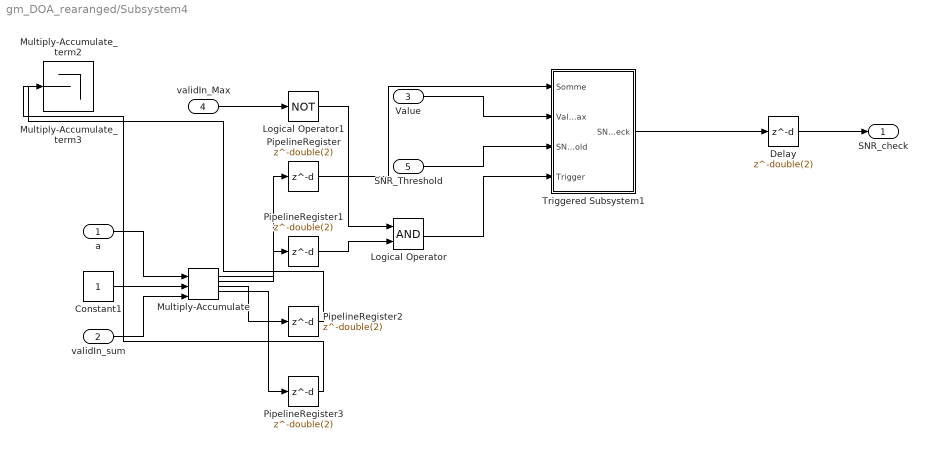
== system gm_DOA_rearanged/Subsystem4 ==
  a : Inport  OutDataTypeStr=fixdt(1, 27, 8)  PortDimensions=1  SampleTime=3.90625e-06
  validIn_sum : Inport  Port=2  OutDataTypeStr=boolean  PortDimensions=1  SampleTime=3.90625e-06
  " Value" : Inport  Port=3  OutDataTypeStr=fixdt(1, 27, 8)  PortDimensions=1  SampleTime=3.90625e-06
  validIn_Max : Inport  Port=4  OutDataTypeStr=boolean  PortDimensions=1  SampleTime=3.90625e-06
  SNR_Threshold : Inport  Port=5  OutDataTypeStr=uint16  PortDimensions=1  SampleTime=3.90625e-06
  Constant1 : Constant  OutDataTypeStr=fixdt(1, 27, 8)  SampleTime=3.90625e-06
  Delay : Delay  DelayLength=double(2)  InitialCondition=0  SampleTime=3.90625e-06
  Logical Operator : Logic  AllPortsSameDT=off  OutDataTypeStr=boolean  SampleTime=3.90625e-06
  Logical Operator1 : Logic  Operator=NOT  Inputs=1  AllPortsSameDT=off  OutDataTypeStr=boolean  SampleTime=3.90625e-06
  Multiply-Accumulate : hdlsllib/HDL Operations/Multiply-Accumulate  opMode=Streaming - using Number of Samples  initValueSetting=Dialog  initValue=0  initValueSetting2=Dialog  initValue2=0  initValueSetting3=Dialog  initValue3=0  num_samples=256  RndMeth2=Floor  RndMeth3=Floor  datatype2=Inherit: Inherit via back propagation  datatype3=fixdt(1, 27, 8)  validOut=on  endInandOut=on  startOut=on  countOut=on  dim=-1  DoSatur=off  parallel=off
      settings: SourceProductBaseCode=SL
  Multiply-Accumulate_term2 : Terminator
  Multiply-Accumulate_term3 : Terminator
  PipelineRegister : Delay  DelayLength=double(2)  InitialCondition=0  SampleTime=3.90625e-06
  PipelineRegister1 : Delay  DelayLength=double(2)  InitialCondition=0  SampleTime=3.90625e-06
  PipelineRegister2 : Delay  DelayLength=double(2)  InitialCondition=1  SampleTime=3.90625e-06
  PipelineRegister3 : Delay  DelayLength=double(2)  InitialCondition=0  SampleTime=3.90625e-06
  Triggered Subsystem1 : Subsystem
  SNR_check : Outport
  wires:
  a/1 -> Multiply-Accumulate/1
  validIn_sum/1 -> Multiply-Accumulate/3
  " Value"/1 -> Triggered Subsystem1/2(" Valeur Max")
  validIn_Max/1 -> Logical Operator1/1
  SNR_Threshold/1 -> Triggered Subsystem1/3(SNR_Threshold)
  Constant1/1 -> Multiply-Accumulate/2
  Delay/1 -> SNR_check/1
  Logical Operator/1 -> Triggered Subsystem1/4(Trigger)
  Logical Operator1/1 -> Logical Operator/1
  PipelineRegister/1 -> Triggered Subsystem1/1(Somme)
  PipelineRegister1/1 -> Logical Operator/2
  PipelineRegister2/1 -> Multiply-Accumulate_term2/1
  PipelineRegister3/1 -> Multiply-Accumulate_term3/1
  Triggered Subsystem1/1(SNR check) -> Delay/1
  Multiply-Accumulate/1 -> PipelineRegister/1
  Multiply-Accumulate/2 -> PipelineRegister1/1
  Multiply-Accumulate/3 -> PipelineRegister2/1
  Multiply-Accumulate/4 -> PipelineRegister3/1

== system gm_DOA_rearanged/Maximum Hydro 1/Sample and Hold ==
  In : Inport  OutDataTypeStr=fixdt(1, 27, 8)
  Trigger : TriggerPort  TriggerType=falling  VariantControl=(inherit)  OutDataTypeStr=boolean
  " " : Outport  InitialOutput=0
  wires:
  In/1 -> " "/1

== system gm_DOA_rearanged/Maximum Hydro 1/Sample and Hold4 ==
  In : Inport  OutDataTypeStr=fixdt(1, 29, 26)
  Trigger : TriggerPort  TriggerType=falling  VariantControl=(inherit)  OutDataTypeStr=boolean
  " " : Outport  InitialOutput=0
  wires:
  In/1 -> " "/1

== system gm_DOA_rearanged/Maximum Hydro 1/Sample and Hold5 ==
  In : Inport  OutDataTypeStr=fixdt(1, 29, 26)
  Trigger : TriggerPort  TriggerType=falling  VariantControl=(inherit)  OutDataTypeStr=boolean
  " " : Outport  InitialOutput=0
  wires:
  In/1 -> " "/1

== system gm_DOA_rearanged/Maximum Hydro 1/Subsystem ==
  Enable/Reset : Inport  OutDataTypeStr=boolean  PortDimensions=1  SampleTime=3.90625e-06
  Add : Sum  AccumDataTypeStr=fixdt(0, 17, 0)  OutDataTypeStr=fixdt(0, 17, 0)  SampleTime=3.90625e-06
  Data Type Conversion1 : DataTypeConversion  OutDataTypeStr=uint16  RndMeth=Nearest  SampleTime=3.90625e-06
  PipelineRegister : Delay  DelayLength=double(1)  InitialCondition=0  SampleTime=3.90625e-06
  Product2 : Product  Inputs=**  OutDataTypeStr=fixdt(0, 17, 0)  SampleTime=3.90625e-06
  Count : Outport  VectorParamsAs1DForOutWhenUnconnected=off
  wires:
  Enable/Reset/1 -> Add/1, Product2/1
  PipelineRegister/1 -> Count/1, Data Type Conversion1/1
  Data Type Conversion1/1 -> Add/2
  Add/1 -> Product2/2
  Product2/1 -> PipelineRegister/1

== system gm_DOA_rearanged/Maximum Hydro 2/Sample and Hold ==
  In : Inport  OutDataTypeStr=fixdt(1, 27, 8)
  Trigger : TriggerPort  TriggerType=falling  VariantControl=(inherit)  OutDataTypeStr=boolean
  " " : Outport  InitialOutput=0
  wires:
  In/1 -> " "/1

== system gm_DOA_rearanged/Maximum Hydro 2/Sample and Hold4 ==
  In : Inport  OutDataTypeStr=fixdt(1, 29, 26)
  Trigger : TriggerPort  TriggerType=falling  VariantControl=(inherit)  OutDataTypeStr=boolean
  " " : Outport  InitialOutput=0
  wires:
  In/1 -> " "/1

== system gm_DOA_rearanged/Maximum Hydro 2/Sample and Hold5 ==
  In : Inport  OutDataTypeStr=fixdt(1, 29, 26)
  Trigger : TriggerPort  TriggerType=falling  VariantControl=(inherit)  OutDataTypeStr=boolean
  " " : Outport  InitialOutput=0
  wires:
  In/1 -> " "/1

== system gm_DOA_rearanged/Maximum Hydro 2/Subsystem ==
  Enable/Reset : Inport  OutDataTypeStr=boolean  PortDimensions=1  SampleTime=3.90625e-06
  Add : Sum  AccumDataTypeStr=fixdt(0, 17, 0)  OutDataTypeStr=fixdt(0, 17, 0)  SampleTime=3.90625e-06
  Data Type Conversion1 : DataTypeConversion  OutDataTypeStr=uint16  RndMeth=Nearest  SampleTime=3.90625e-06
  PipelineRegister : Delay  DelayLength=double(1)  InitialCondition=0  SampleTime=3.90625e-06
  Product2 : Product  Inputs=**  OutDataTypeStr=fixdt(0, 17, 0)  SampleTime=3.90625e-06
  Count : Outport  VectorParamsAs1DForOutWhenUnconnected=off
  wires:
  Enable/Reset/1 -> Add/1, Product2/1
  PipelineRegister/1 -> Count/1, Data Type Conversion1/1
  Data Type Conversion1/1 -> Add/2
  Add/1 -> Product2/2
  Product2/1 -> PipelineRegister/1

== system gm_DOA_rearanged/Maximum Hydro 3/Sample and Hold ==
  In : Inport  OutDataTypeStr=fixdt(1, 27, 8)
  Trigger : TriggerPort  TriggerType=falling  VariantControl=(inherit)  OutDataTypeStr=boolean
  " " : Outport  InitialOutput=0
  wires:
  In/1 -> " "/1

== system gm_DOA_rearanged/Maximum Hydro 3/Sample and Hold4 ==
  In : Inport  OutDataTypeStr=fixdt(1, 29, 26)
  Trigger : TriggerPort  TriggerType=falling  VariantControl=(inherit)  OutDataTypeStr=boolean
  " " : Outport  InitialOutput=0
  wires:
  In/1 -> " "/1

== system gm_DOA_rearanged/Maximum Hydro 3/Sample and Hold5 ==
  In : Inport  OutDataTypeStr=fixdt(1, 29, 26)
  Trigger : TriggerPort  TriggerType=falling  VariantControl=(inherit)  OutDataTypeStr=boolean
  " " : Outport  InitialOutput=0
  wires:
  In/1 -> " "/1

== system gm_DOA_rearanged/Maximum Hydro 3/Subsystem ==
  Enable/Reset : Inport  OutDataTypeStr=boolean  PortDimensions=1  SampleTime=3.90625e-06
  Add : Sum  AccumDataTypeStr=fixdt(0, 17, 0)  OutDataTypeStr=fixdt(0, 17, 0)  SampleTime=3.90625e-06
  Data Type Conversion1 : DataTypeConversion  OutDataTypeStr=uint16  RndMeth=Nearest  SampleTime=3.90625e-06
  PipelineRegister : Delay  DelayLength=double(1)  InitialCondition=0  SampleTime=3.90625e-06
  Product2 : Product  Inputs=**  OutDataTypeStr=fixdt(0, 17, 0)  SampleTime=3.90625e-06
  Count : Outport  VectorParamsAs1DForOutWhenUnconnected=off
  wires:
  Enable/Reset/1 -> Add/1, Product2/1
  PipelineRegister/1 -> Count/1, Data Type Conversion1/1
  Data Type Conversion1/1 -> Add/2
  Add/1 -> Product2/2
  Product2/1 -> PipelineRegister/1

== system gm_DOA_rearanged/Maximum Hydro Ref/Sample and Hold ==
  In : Inport  OutDataTypeStr=fixdt(1, 27, 8)
  Trigger : TriggerPort  TriggerType=falling  VariantControl=(inherit)  OutDataTypeStr=boolean
  " " : Outport  InitialOutput=0
  wires:
  In/1 -> " "/1

== system gm_DOA_rearanged/Maximum Hydro Ref/Sample and Hold1 ==
  In : Inport  OutDataTypeStr=fixdt(0, 17, 0)
  Trigger : TriggerPort  TriggerType=falling  VariantControl=(inherit)  OutDataTypeStr=boolean
  " " : Outport  InitialOutput=0
  wires:
  In/1 -> " "/1

== system gm_DOA_rearanged/Maximum Hydro Ref/Sample and Hold2 ==
  In : Inport  OutDataTypeStr=fixdt(1, 27, 8)
  Trigger : TriggerPort  TriggerType=falling  VariantControl=(inherit)  OutDataTypeStr=boolean
  " " : Outport  InitialOutput=0
  wires:
  In/1 -> " "/1

== system gm_DOA_rearanged/Maximum Hydro Ref/Sample and Hold3 ==
  In : Inport  OutDataTypeStr=fixdt(0, 17, 0)
  Trigger : TriggerPort  TriggerType=falling  VariantControl=(inherit)  OutDataTypeStr=boolean
  " " : Outport  InitialOutput=0
  wires:
  In/1 -> " "/1

== system gm_DOA_rearanged/Maximum Hydro Ref/Sample and Hold4 ==
  In : Inport  OutDataTypeStr=fixdt(1, 29, 26)
  Trigger : TriggerPort  TriggerType=falling  VariantControl=(inherit)  OutDataTypeStr=boolean
  " " : Outport  InitialOutput=0
  wires:
  In/1 -> " "/1

== system gm_DOA_rearanged/Maximum Hydro Ref/Sample and Hold5 ==
  In : Inport  OutDataTypeStr=fixdt(1, 29, 26)
  Trigger : TriggerPort  TriggerType=falling  VariantControl=(inherit)  OutDataTypeStr=boolean
  " " : Outport  InitialOutput=0
  wires:
  In/1 -> " "/1

== system gm_DOA_rearanged/Maximum Hydro Ref/Subsystem ==
  Enable/Reset : Inport  OutDataTypeStr=boolean  PortDimensions=1  SampleTime=3.90625e-06
  Add : Sum  AccumDataTypeStr=fixdt(0, 17, 0)  OutDataTypeStr=fixdt(0, 17, 0)  SampleTime=3.90625e-06
  Data Type Conversion1 : DataTypeConversion  OutDataTypeStr=uint16  RndMeth=Nearest  SampleTime=3.90625e-06
  PipelineRegister : Delay  DelayLength=double(1)  InitialCondition=0  SampleTime=3.90625e-06
  Product2 : Product  Inputs=**  OutDataTypeStr=fixdt(0, 17, 0)  SampleTime=3.90625e-06
  Count : Outport  VectorParamsAs1DForOutWhenUnconnected=off
  wires:
  Enable/Reset/1 -> Add/1, Product2/1
  PipelineRegister/1 -> Count/1, Data Type Conversion1/1
  Data Type Conversion1/1 -> Add/2
  Add/1 -> Product2/2
  Product2/1 -> PipelineRegister/1

== system gm_DOA_rearanged/Signal Trigger/Fenetrage ==
  Valid_in : Inport  OutDataTypeStr=boolean  PortDimensions=1  SampleTime=3.90625e-06
  Enable : Inport  Port=2  OutDataTypeStr=boolean  PortDimensions=1  SampleTime=3.90625e-06
  Constant : Constant  Value=0  OutDataTypeStr=uint16  SampleTime=1/Sampling_rate
  Direct Lookup Table (n-D) : LookupNDDirect  NumberOfTableDimensions=1  Table=Coeff_han  DiagnosticForOutOfRangeInput=Error  TableMin=[0]  TableDataTypeStr=fixdt(0,9,8)
  Subsystem : Subsystem
  Switch : Switch  Threshold=FFT_LENGTH  OutMin=[0]  OutMax=[511]  OutDataTypeStr=uint16
  coeff : Outport
  wires:
  Valid_in/1 -> Subsystem/1(Reset)
  Enable/1 -> Subsystem/2(Enable)
  Constant/1 -> Switch/1
  Direct Lookup Table (n-D)/1 -> coeff/1
  Subsystem/1(Count) -> Switch/3, Switch/2
  Switch/1 -> Direct Lookup Table (n-D)/1

== system gm_DOA_rearanged/Signal Trigger/Sample and Hold ==
  In : Inport  OutDataTypeStr=boolean
  Trigger : TriggerPort  VariantControl=(inherit)  OutDataTypeStr=boolean
  " " : Outport  InitialOutput=0
  wires:
  In/1 -> " "/1

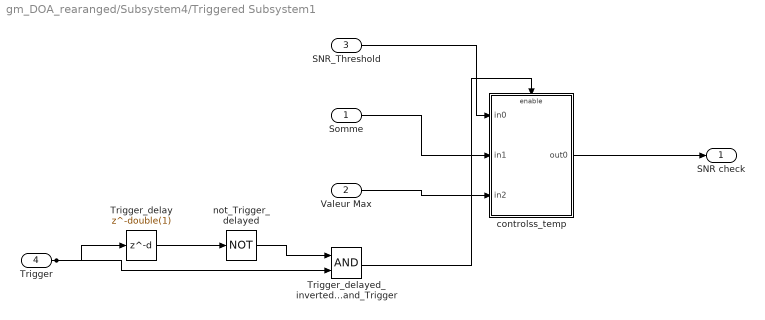
== system gm_DOA_rearanged/Subsystem4/Triggered Subsystem1 ==
  Somme : Inport  OutDataTypeStr=fixdt(1, 27, 8)  PortDimensions=1  SampleTime=3.90625e-06
  " Valeur Max" : Inport  Port=2  OutDataTypeStr=fixdt(1, 27, 8)  PortDimensions=1  SampleTime=3.90625e-06
  SNR_Threshold : Inport  Port=3  OutDataTypeStr=uint16  PortDimensions=1  SampleTime=3.90625e-06
  Trigger : Inport  Port=4  OutDataTypeStr=boolean  SampleTime=3.90625e-06
  Trigger_delay : Delay  DelayLength=double(1)  InitialCondition=1
  Trigger_delayed_inverted_and_Trigger : Logic  AllPortsSameDT=off  OutDataTypeStr=boolean  SampleTime=3.90625e-06
  controlss_temp : Subsystem
  not_Trigger_delayed : Logic  Operator=NOT  Inputs=1  AllPortsSameDT=off  OutDataTypeStr=boolean  SampleTime=3.90625e-06
  SNR check : Outport  InitialOutput=0  VectorParamsAs1DForOutWhenUnconnected=off
  wires:
  Trigger/1 -> Trigger_delayed_inverted_and_Trigger/2, Trigger_delay/1
  Somme/1 -> controlss_temp/2(in1)
  " Valeur Max"/1 -> controlss_temp/3(in2)
  SNR_Threshold/1 -> controlss_temp/1(in0)
  controlss_temp/1(out0) -> SNR check/1
  Trigger_delay/1 -> not_Trigger_delayed/1
  not_Trigger_delayed/1 -> Trigger_delayed_inverted_and_Trigger/1
  Trigger_delayed_inverted_and_Trigger/1 -> controlss_temp/Enable

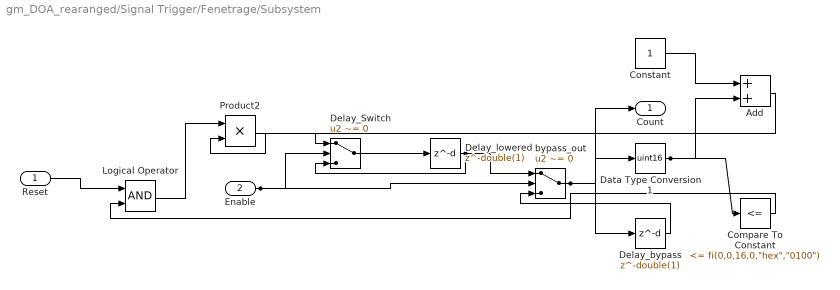
== system gm_DOA_rearanged/Signal Trigger/Fenetrage/Subsystem ==
  Reset : Inport  OutDataTypeStr=boolean  PortDimensions=1  SampleTime=3.90625e-06
  Enable : Inport  Port=2  OutDataTypeStr=boolean  PortDimensions=1  SampleTime=3.90625e-06
  Add : Sum  AccumDataTypeStr=fixdt(0, 17, 0)  OutDataTypeStr=fixdt(0, 17, 0)  SampleTime=3.90625e-06
  Compare To Constant : simulink/Logic and Bit Operations/Compare To Constant  relop=<=  const="fi(0,0,16,0,\"hex\",\"0100\")"  OutDataTypeStr=boolean
  Constant : Constant  OutDataTypeStr=uint16  SampleTime=3.90625e-06
  Data Type Conversion1 : DataTypeConversion  OutDataTypeStr=uint16  RndMeth=Nearest  SampleTime=3.90625e-06
  Delay_Switch : Switch  Criteria=u2 ~= 0  Threshold=double(0)  OutDataTypeStr=uint16  SampleTime=3.90625e-06
  Delay_bypass : Delay  DelayLength=double(1)  InitialCondition=0  SampleTime=3.90625e-06
  Delay_lowered : Delay  DelayLength=double(1)  InitialCondition=0  SampleTime=3.90625e-06
  Logical Operator : Logic  AllPortsSameDT=off  OutDataTypeStr=boolean  SampleTime=3.90625e-06
  Product2 : Product  Inputs=**  OutDataTypeStr=uint16  SampleTime=3.90625e-06
  bypass_out : Switch  Criteria=u2 ~= 0  Threshold=double(0)  OutDataTypeStr=uint16  SampleTime=3.90625e-06
  Count : Outport  VectorParamsAs1DForOutWhenUnconnected=off
  wires:
  Reset/1 -> Logical Operator/1
  Enable/1 -> bypass_out/2, Delay_Switch/2
  Add/1 -> Product2/2
  Compare To Constant/1 -> Logical Operator/2
  Constant/1 -> Add/1
  Data Type Conversion1/1 -> Compare To Constant/1, Add/2
  bypass_out/1 -> Data Type Conversion1/1, Delay_bypass/1, Count/1
  Logical Operator/1 -> Product2/1
  Product2/1 -> Delay_Switch/1
  Delay_lowered/1 -> bypass_out/1, Delay_Switch/3
  Delay_Switch/1 -> Delay_lowered/1
  Delay_bypass/1 -> bypass_out/3

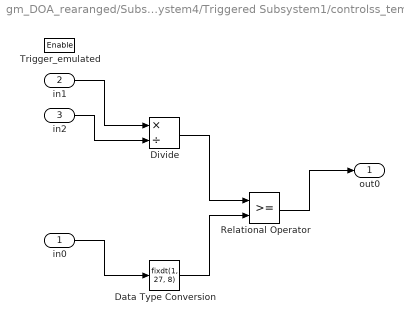
== system gm_DOA_rearanged/Subsystem4/Triggered Subsystem1/controlss_temp ==
  in0 : Inport  OutDataTypeStr=uint16  SampleTime=3.90625e-06
  in1 : Inport  Port=2  OutDataTypeStr=fixdt(1, 27, 8)  SampleTime=3.90625e-06
  in2 : Inport  Port=3  OutDataTypeStr=fixdt(1, 27, 8)  SampleTime=3.90625e-06
  Trigger_emulated : EnablePort  OutDataTypeStr=boolean
  Data Type Conversion : DataTypeConversion  OutDataTypeStr=fixdt(1, 27, 8)  SampleTime=3.90625e-06
  Divide : Product  Inputs=*/  OutDataTypeStr=fixdt(1, 27, 0)  RndMeth=Zero  SaturateOnIntegerOverflow=on  SampleTime=3.90625e-06
  Relational Operator : RelationalOperator  OutDataTypeStr=boolean  SampleTime=3.90625e-06  RndMeth=Nearest
  out0 : Outport  OutDataTypeStr=boolean  InitialOutput=0
  wires:
  Data Type Conversion/1 -> Relational Operator/2
  Divide/1 -> Relational Operator/1
  Relational Operator/1 -> out0/1
  in0/1 -> Data Type Conversion/1
  in1/1 -> Divide/1
  in2/1 -> Divide/2
